simulink model "PLL_FOC_33AK512MC510_MCLV_48V_solution"  (R2025b)
settings: Solver=FixedStepDiscrete  StartTime=0.0  StopTime=3  FixedStep=50e-6  RelTol=1e-3  EnableMultiTasking=on
values from neighbouring files (symbols this model uses):
  a_ho = 2*pi*f_ho_lpf*Ts    [foc_ctrl_params.m]
  f_ho = 25    [foc_ctrl_params.m]
  I_align = 3.0    (= 3)    [foc_ctrl_params.m]
  I_start = 3.0    (= 3)    [foc_ctrl_params.m]
  iq_max = 4    [foc_ctrl_params.m]
  Kp_i = Lc*wc_i    [foc_ctrl_params.m]
  Kp_w = J*wc_w/(p*Kt)    [foc_ctrl_params.m]
  Lc = Ls    [foc_ctrl_params.m]
  psi = 9.2386e-3    (= 0.0092386)    [params_ACT_57BLF02.m]
  t_adc = 1.0    (= 1)    [foc_ctrl_params.m]
  t_align = 0.15    [foc_ctrl_params.m]
  t_ho = t_adc + t_align + t_ramp    (= 1.6)    [foc_ctrl_params.m]
  t_ramp = 0.45    [foc_ctrl_params.m]    (also in obs_params.m = 0.6)
  Ts = 1/PWM_frequency    (= 5e-05)    [obs_params.m]    (also in params_ACT_57BLF02.m)
  Tss = 10*Ts    [foc_ctrl_params.m]
  Vmax = Vdc/sqrt(3)    [foc_ctrl_params.m]
  wref = 2*pi*30    (= 188.495559215)    [foc_ctrl_params.m]
undefined symbols (not defined in the file or in its folder): A0, A4, ADC, B0, C10, C11, C12, C13, C14, C15, C2, C3, C4, C5, CND4max, D0, D1, D10, D2, D3, D4, D5, D6, D9, DiscIntNeverNeededParam, Max, MaxPer, ms, NumBits1, NumBits2, P1, P17, P20, P35, P36, P37, P38, P43, P44, P45, P46, P47, P48, P49, P50, P51, P52, P54, P55, P58, P59, Pin, pll, PWM1_Trg1, Resol, s, us
libraries: simulink x30, MCHP_Blockset x20, embmathops x1
(part 3 of 5)

== system PLL_FOC_33AK512MC510_MCLV_48V_solution/Bipolar to Unipolar PWM input set for input in [0 1] ==
  note: Output default value is 0.5 on all 3 channels enabling current bias estimator
  In [-1 1] : Inport
  Enable : EnablePort
  Bias : Bias  Bias=0.5  SaturateOnIntegerOverflow=off
  Gain : Gain  Gain=0.5
  Out [0 1] : Outport  OutputWhenDisabled=reset  InitialOutput=[0.5 0.5 0.5]'
  wires:
  Bias/1 -> Out [0 1]/1
  Gain/1 -> Bias/1
  In [-1 1]/1 -> Gain/1

== system PLL_FOC_33AK512MC510_MCLV_48V_solution/Clarke ==
  note: $\textbf{Clarke transform}\;(abc \rightarrow \alpha\beta)\\\alpha = \frac{2}{3}\!\left(a-\frac{b}{2}-\frac{c}{2}\right),\quad \beta = \frac{b-c}{\sqrt{3}}\\\text{amplitude-invariant, } \alpha \text{ on phase-}a\text{ axis, } \beta \text{ at } +90^{\circ}.\\\text{If } a+b+c=0:\quad \alpha=a,\;\; \beta=\frac{a+2b}{\sqrt{3}}\;\text{(2-input form used here).}$
  ab(c) : Inport
  C1 : Gain  Gain=[1/sqrt(3) 2/sqrt(3)]  Multiplication=Matrix(K*u)  OutDataTypeStr=Inherit: Same as input  ParamDataTypeStr=Inherit: Same as input
  Mux : Mux  Inputs=2
  Selector : Selector  InputPortWidth=2  IndexOptions=Index vector (dialog)  Indices=[1]  OutputSizes=1
  alphabeta : Outport  VectorParamsAs1DForOutWhenUnconnected=off
  wires:
  C1/1 -> Mux/2
  Selector/1 -> Mux/1
  Mux/1 -> alphabeta/1
  ab(c)/1 -> C1/1, Selector/1

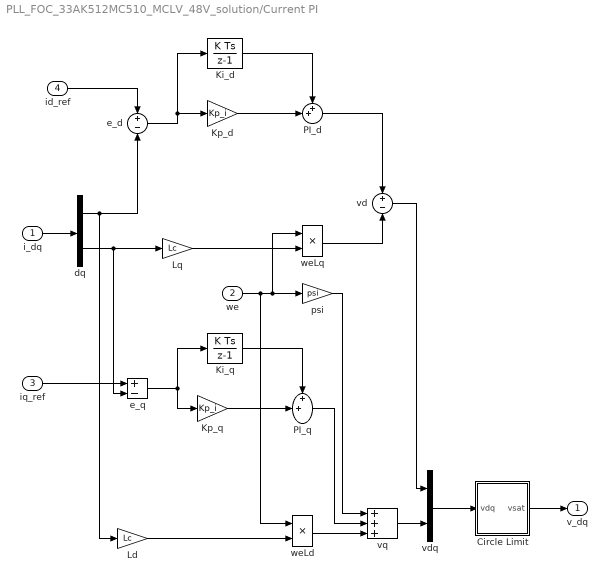
== system PLL_FOC_33AK512MC510_MCLV_48V_solution/Current PI ==
  i_dq : Inport
  we : Inport  Port=2
  iq_ref : Inport  Port=3
  id_ref : Inport  Port=4
  Circle Limit : Subsystem
  Ki_d : DiscreteIntegrator  gainval=Ki_i  SampleTime=Ts  LimitOutput=on  UpperSaturationLimit=Vmax  LowerSaturationLimit=-Vmax  ICPrevOutput=DiscIntNeverNeededParam  ICPrevScaledInput=DiscIntNeverNeededParam
  Ki_q : DiscreteIntegrator  gainval=Ki_i  SampleTime=Ts  LimitOutput=on  UpperSaturationLimit=Vmax  LowerSaturationLimit=-Vmax  ICPrevOutput=DiscIntNeverNeededParam  ICPrevScaledInput=DiscIntNeverNeededParam
  Kp_d : Gain  Gain=Kp_i
  Kp_q : Gain  Gain=Kp_i
  Ld : Gain  Gain=Lc
  Lq : Gain  Gain=Lc
  PI_d : Sum  Inputs=++|
  PI_q : Sum  Inputs=++|
  dq : Demux  Outputs=2
  e_d : Sum  Inputs=+-
  e_q : Sum  Inputs=+-
  psi : Gain  Gain=psi
  vd : Sum  Inputs=+-
  vdq : Mux  Inputs=2
  vq : Sum  Inputs=+++
  weLd : Product  Inputs=**
  weLq : Product  Inputs=**
  v_dq : Outport
  wires:
  i_dq/1 -> dq/1
  dq/2 -> e_q/2, Lq/1
  id_ref/1 -> e_d/1
  iq_ref/1 -> e_q/1
  dq/1 -> e_d/2, Ld/1
  e_q/1 -> Kp_q/1, Ki_q/1
  e_d/1 -> Kp_d/1, Ki_d/1
  Lq/1 -> weLq/2
  Ld/1 -> weLd/2
  weLq/1 -> vd/2
  Ki_d/1 -> PI_d/1
  Kp_d/1 -> PI_d/2
  we/1 -> psi/1, weLq/1, weLd/1
  Ki_q/1 -> PI_q/1
  Kp_q/1 -> PI_q/2
  PI_d/1 -> vd/1
  psi/1 -> vq/1
  PI_q/1 -> vq/2
  Circle Limit/1(vsat) -> v_dq/1
  weLd/1 -> vq/3
  vd/1 -> vdq/1
  vq/1 -> vdq/2
  vdq/1 -> Circle Limit/1(vdq)

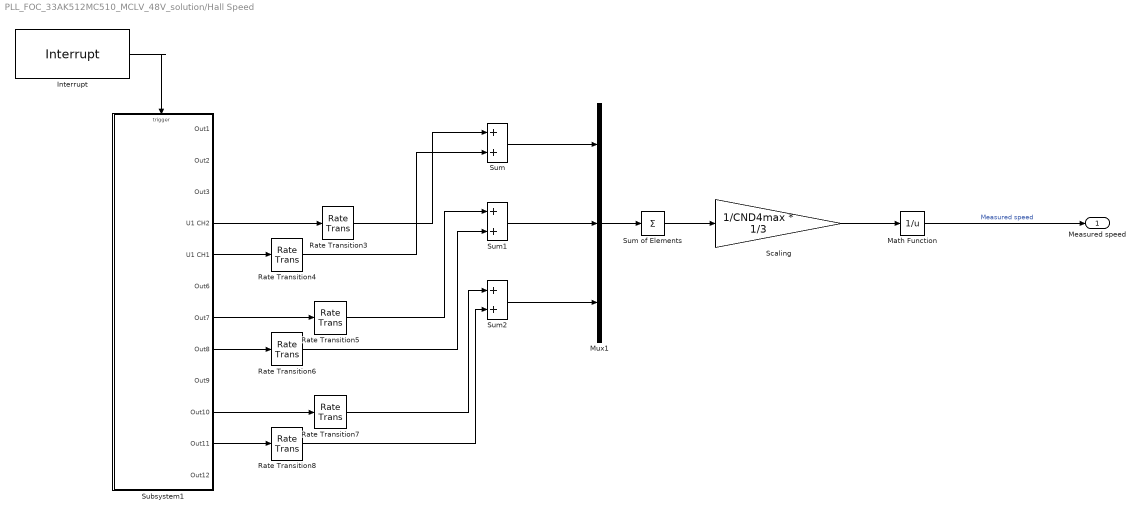
== system PLL_FOC_33AK512MC510_MCLV_48V_solution/Hall Speed ==
  Interrupt : MCHP_Blockset/System Functions/Interrupt  Interruption_TXT=CND  InterruptionLongDesc=Change Notification - D  IntPriority=5  IntPriority_Info=Priority 5 (set by PLL_FOC_33AK512MC510_MCLV_48V_solution/Hall Speed/Subsystem1/Change Notification1)  StartupExecute=off  ClearActionState=CND:if:CNDIF:0=1  Status=OK  MCHP_MASTERLINK=PLL_FOC_33AK512MC510_MCLV_48V_solution/BOARD MCLV-48V-300W dsPIC33AK512MC510 MC DIM1/Microchip Master  FPUNoSave=on  Triggered_Sub_TimeSource=is derived from model base rate  TrigsPeriod=0  TIMER_Resolution_TXT="Resol: 0.01(us)  -  MaxPer: 0.655(ms)"  Info=0  SS_ASYNCHRONOUS_INTERRUPT=1  SS_TIMESOURCE=1  SS_AsyncTimerRes=-1  SS_AsyncTaskPriority=5  SS_ARCH=16
      settings: SourceProductName=MPLAB Device Blocks for Simulink
  Math Function : Math  Operator=reciprocal  OutDataTypeStr=single
  Mux1 : Mux  Inputs=3
  Rate Transition3 : RateTransition  Deterministic=off  OutPortSampleTime=50e-6
  Rate Transition{4..8} (5 alike) : RateTransition  Deterministic=off
  Scaling : Gain  Gain=1/CND4max * 1/3  OutDataTypeStr=single
  Subsystem1 : Subsystem
  Sum : Sum  SaturateOnIntegerOverflow=on
  Sum of Elements : Sum  Inputs=+
  Sum1 : Sum  SaturateOnIntegerOverflow=on
  Sum2 : Sum  SaturateOnIntegerOverflow=on
  Measured speed : Outport
  wires:
  Subsystem1/5(U1 CH1) -> Rate Transition4/1
  Sum/1 -> Mux1/1
  Rate Transition5/1 -> Sum1/1
  Rate Transition8/1 -> Sum2/2
  Rate Transition3/1 -> Sum/1
  Interrupt/1 -> Subsystem1/Trigger
  Subsystem1/8(Out8) -> Rate Transition6/1
  Scaling/1 -> Math Function/1
  Sum of Elements/1 -> Scaling/1
  Sum1/1 -> Mux1/2
  Rate Transition6/1 -> Sum1/2
  Sum2/1 -> Mux1/3
  Subsystem1/11(Out11) -> Rate Transition8/1
  Rate Transition7/1 -> Sum2/1
  Mux1/1 -> Sum of Elements/1
  Subsystem1/7(Out7) -> Rate Transition5/1
  Subsystem1/10(Out10) -> Rate Transition7/1
  Subsystem1/4(U1 CH2) -> Rate Transition3/1
  Rate Transition4/1 -> Sum/2
  Math Function/1 -> Measured speed/1  "Measured speed"

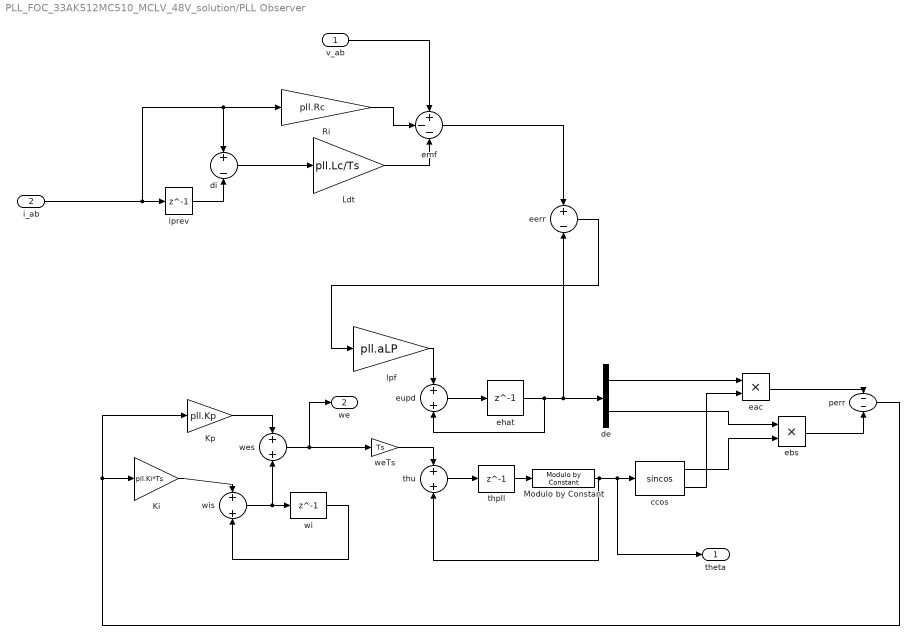
== system PLL_FOC_33AK512MC510_MCLV_48V_solution/PLL Observer ==
  v_ab : Inport
  i_ab : Inport  Port=2
  Ki : Gain  Gain=pll.Ki*Ts
  Kp : Gain  Gain=pll.Kp
  Ldt : Gain  Gain=pll.Lc/Ts
  Modulo by Constant : embmathops/Modulo by Constant  Denominator=2*pi  SimulateUsing=Code generation
      settings: LibrarySourceBlock=embeddedMathLib/Modulo by Constant
  Ri : Gain  Gain=pll.Rc
  ccos : Trigonometry  Operator=sincos
  de : Demux  Outputs=2
  di : Sum  Inputs=+-
  eac : Product  Inputs=**
  ebs : Product  Inputs=**
  eerr : Sum  Inputs=+-
  ehat : Delay  DelayLength=1  InitialCondition=0  SampleTime=Ts
  emf : Sum  Inputs=+--
  eupd : Sum
  iprev : Delay  DelayLength=1  InitialCondition=0  SampleTime=Ts
  lpf : Gain  Gain=pll.aLP
  perr : Sum  Inputs=--
  thpll : Delay  DelayLength=1  InitialCondition=0  SampleTime=Ts
  thu : Sum
  weTs : Gain  Gain=Ts
  wes : Sum
  wi : Delay  DelayLength=1  InitialCondition=0  SampleTime=Ts
  wis : Sum
  theta : Outport  OutDataTypeStr=single
  we : Outport  Port=2  OutDataTypeStr=single
  wires:
  i_ab/1 -> di/1, Ri/1, iprev/1
  wis/1 -> wes/2, wi/1
  iprev/1 -> di/2
  Ri/1 -> emf/2
  wes/1 -> weTs/1, we/1
  di/1 -> Ldt/1
  de/1 -> eac/1
  wi/1 -> wis/2
  lpf/1 -> eupd/1
  ebs/1 -> perr/2
  weTs/1 -> thu/1
  v_ab/1 -> emf/1
  Ldt/1 -> emf/3
  Kp/1 -> wes/1
  eupd/1 -> ehat/1
  thu/1 -> thpll/1
  emf/1 -> eerr/1
  ehat/1 -> de/1, eerr/2, eupd/2
  thpll/1 -> Modulo by Constant/1
  eerr/1 -> lpf/1
  de/2 -> ebs/1
  ccos/2 -> eac/2
  ccos/1 -> ebs/2
  eac/1 -> perr/1
  perr/1 -> Kp/1, Ki/1
  Ki/1 -> wis/1
  Modulo by Constant/1 -> thu/2, theta/1, ccos/1

== system PLL_FOC_33AK512MC510_MCLV_48V_solution/Park meas ==
  i_ab : Inport
  theta : Inport  Port=2
  ab : Demux  Outputs=2
  ac : Product  Inputs=**
  as : Product  Inputs=**
  bc : Product  Inputs=**
  bs : Product  Inputs=**
  cos : Trigonometry  Operator=cos
  dq : Mux  Inputs=2
  id : Sum
  iq : Sum  Inputs=-+
  sin : Trigonometry
  i_dq : Outport
  wires:
  i_ab/1 -> ab/1
  sin/1 -> as/2, bs/2
  theta/1 -> cos/1, sin/1
  ab/2 -> bs/1, bc/1
  ab/1 -> ac/1, as/1
  cos/1 -> ac/2, bc/2
  ac/1 -> id/1
  bs/1 -> id/2
  as/1 -> iq/1
  bc/1 -> iq/2
  id/1 -> dq/1
  iq/1 -> dq/2
  dq/1 -> i_dq/1

== system PLL_FOC_33AK512MC510_MCLV_48V_solution/Speed PI ==
  note: BUMPLESS I-f -> CL HANDOVER
      | Ki is held reset (IC = external) while hold = 1.
      | IC = LPF(iq_meas) - Kp_w*e  =>  iq_ref is continuous at t_ho.
      | Preload follows I_start automatically (no constant to retune).
  w_ref : Inport
  w_fb : Inport  Port=2
  hold : Inport  Port=3
  iq_meas : Inport  Port=4
  Ki : DiscreteIntegrator  gainval=Ki_w  ExternalReset=level  InitialConditionSource=external  SampleTime=Tss  LimitOutput=on  UpperSaturationLimit=iq_max  LowerSaturationLimit=-iq_max  ICPrevOutput=DiscIntNeverNeededParam  ICPrevScaledInput=DiscIntNeverNeededParam
  Kp : Gain  Gain=Kp_w
  err : Sum  Inputs=+-
  ic : Sum  Inputs=+-
  iqf : DiscreteTransferFcn  Numerator=[a_ho 0]  Denominator=[1 -(1-a_ho)]  SampleTime=Ts
  lim : Saturate  UpperLimit=iq_max  LowerLimit=-iq_max
  sum : Sum
  iq_ref : Outport
  wires:
  w_ref/1 -> err/1
  w_fb/1 -> err/2
  err/1 -> Ki/1, Kp/1
  hold/1 -> Ki/2
  Kp/1 -> sum/1, ic/2
  Ki/1 -> sum/2
  sum/1 -> lim/1
  lim/1 -> iq_ref/1
  iq_meas/1 -> iqf/1
  iqf/1 -> ic/1
  ic/1 -> Ki/3

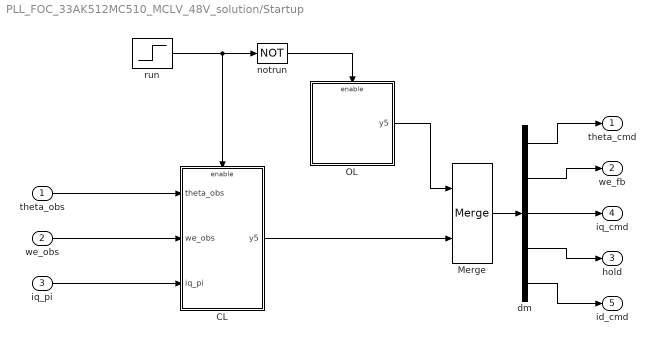
== system PLL_FOC_33AK512MC510_MCLV_48V_solution/Startup ==
  theta_obs : Inport
  we_obs : Inport  Port=2
  iq_pi : Inport  Port=3
  CL : Subsystem  TreatAsAtomicUnit=on
  Merge : Merge
  OL : Subsystem  TreatAsAtomicUnit=on
  dm : Demux  Outputs=5
  notrun : Logic  Operator=NOT  AllPortsSameDT=off  OutDataTypeStr=boolean
  run : Step  Time=t_ho  SampleTime=Ts
  theta_cmd : Outport
  we_fb : Outport  Port=2
  hold : Outport  Port=3
  iq_cmd : Outport  Port=4
  id_cmd : Outport  Port=5
  wires:
  theta_obs/1 -> CL/1(theta_obs)
  notrun/1 -> OL/Enable
  run/1 -> CL/Enable, notrun/1
  dm/1 -> theta_cmd/1
  OL/1(y5) -> Merge/1
  we_obs/1 -> CL/2(we_obs)
  iq_pi/1 -> CL/3(iq_pi)
  CL/1(y5) -> Merge/2
  Merge/1 -> dm/1
  dm/2 -> we_fb/1
  dm/3 -> iq_cmd/1
  dm/4 -> hold/1
  dm/5 -> id_cmd/1

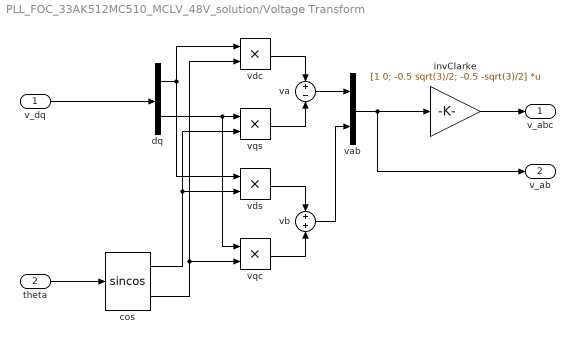
== system PLL_FOC_33AK512MC510_MCLV_48V_solution/Voltage Transform ==
  v_dq : Inport  OutDataTypeStr=single
  theta : Inport  Port=2  OutDataTypeStr=single
  cos : Trigonometry  Operator=sincos
  dq : Demux  Outputs=2
  invClarke : Gain  Gain=[1 0; -0.5 sqrt(3)/2; -0.5 -sqrt(3)/2]  Multiplication=Matrix(K*u)
  va : Sum  Inputs=+-
  vab : Mux  Inputs=2
  vb : Sum
  vdc : Product  Inputs=**
  vds : Product  Inputs=**
  vqc : Product  Inputs=**
  vqs : Product  Inputs=**
  v_abc : Outport
  v_ab : Outport  Port=2
  wires:
  v_dq/1 -> dq/1
  theta/1 -> cos/1
  vqs/1 -> va/2
  cos/1 -> vqs/2, vds/2
  dq/1 -> vdc/1, vds/1
  dq/2 -> vqs/1, vqc/1
  cos/2 -> vdc/2, vqc/2
  invClarke/1 -> v_abc/1
  vdc/1 -> va/1
  vds/1 -> vb/1
  vqc/1 -> vb/2
  va/1 -> vab/1
  vb/1 -> vab/2
  vab/1 -> v_ab/1, invClarke/1
